simulink model "Snake_Robot_Head_Control"  (R2023a)
settings: Solver=ode23tb  StartTime=0.0  StopTime=2000  FixedStep=0.001  RelTol=1e-3
values from neighbouring files (symbols this model uses):
  cn = 5    [parameters_Robot_control.m]
  ct = 1    [parameters_Robot_control.m]
undefined symbols (not defined in the file or in its folder): X, Y, Z
libraries: nesl_utility x85, sm_lib x49
(part 3 of 3)

== system Snake_Robot_Head_Control/SnakeRobot/Link8 ==
  Brick Solid : sm_lib/Body Elements/Brick Solid  GraphicAmbientColor=[0.15 0.15 0.15 1.0]  BasedOnType=Mass  BrickDimensions=[180 80 80]  BrickDimensionsUnits=mm  CenterOfMass=[0 0 0]  CenterOfMassUnits=m  GraphicDiffuseColor=[0.5 0.5 0.5]  Density=1000  DensityUnits=kg/m^3  DoExposeReferenceFrame=on  GraphicEmissiveColor=[0.0 0.0 0.0 1.0]  ExportEntireGeometry=off  SerializedFrames=<Frames><Frame><Id>Frame1</Id><Value><Name>nextlink</Name><Origin><Source>GeometricFeature</Source><FeatureName>+x surface</FeatureName></Origin><PrimaryAxis><DefinedDirection>+Z</DefinedDirection><Source>ReferenceFrame</Source><SourceDirection>+Z</SourceDirection><FeatureName></FeatureName></PrimaryAxis><SecondaryAxis><DefinedDirection>+X</DefinedDirection><Source>ReferenceFrame</Source><SourceDirection>+X</SourceDirection><FeatureName></FeatureName></SecondaryAxis></Value></Frame><Frame><Id>Frame2</Id><Value><Name>P_link</Name><Origin><Source>GeometricFeature</Source><FeatureName>-x surface</FeatureName></Origin><PrimaryAxis><DefinedDirection>+Z</DefinedDirection><Source>ReferenceFrame</Source><SourceDirection>+Z</SourceDirection><FeatureName></FeatureName></PrimaryAxis><SecondaryAxis><DefinedDirection>+X</DefinedDirection><Source>ReferenceFrame</Source><SourceDirection>+X</SourceDirection><FeatureName></FeatureName></SecondaryAxis></Value></Frame><Frame><Id>Frame3</Id><Value><Name>F3</Name><Origin><Source>CenterOfMassFrame</Source><FeatureName></FeatureName></Origin><PrimaryAxis><DefinedDirection>+Z</DefinedDirection><Source>ReferenceFrame</Source><SourceDirection>+Z</SourceDirection><FeatureName></FeatureName></PrimaryAxis><SecondaryAxis><DefinedDirection>+X</DefinedDirection><Source>ReferenceFrame</Source><SourceDirection>+X</SourceDirection><FeatureName></FeatureName></SecondaryAxis></Value></Frame></Frames>  MarkerShape=Sphere  MarkerSize=10  GraphicType=FromGeometry  InertiaType=CalculateFromGeometry  Mass=0.9047  MassUnits=kg  MomentsOfInertia=[1 1 1]  MomentsOfInertiaUnits=kg*m^2  GraphicOpacity=1.0  ProductsOfInertia=[0 0 0]  ProductsOfInertiaUnits=kg*m^2  GraphicShininess=75  GraphicSpecularColor=[0.5 0.5 0.5 1.0]  GraphicVisPropType=SimpleVisualProperties
  Constant : Constant  Value=ct
  Constant1 : Constant  Value=cn
  Integrator : Integrator
  MATLAB Function : MATLAB Function  TreatAsAtomicUnit=on
  PS-Simulink Converter : nesl_utility/PS-Simulink Converter  PhysicalDomain=network_engine_domain  SubClassName=ps_output  LeftPortType=input  RightPortType=output  PseudoPeriodic=off  Frequencies=[]  VectorFormat=inherit  Unit=inherit  AffineConversion=off
  PS-Simulink Converter1 : nesl_utility/PS-Simulink Converter  PhysicalDomain=network_engine_domain  SubClassName=ps_output  LeftPortType=input  RightPortType=output  PseudoPeriodic=off  Frequencies=[]  VectorFormat=inherit  Unit=inherit  AffineConversion=off
  PS-Simulink Converter2 : nesl_utility/PS-Simulink Converter  PhysicalDomain=network_engine_domain  SubClassName=ps_output  LeftPortType=input  RightPortType=output  PseudoPeriodic=off  Frequencies=[]  VectorFormat=inherit  Unit=inherit  AffineConversion=off
  Planar Joint : sm_lib/Joints/Planar Joint  JointMode=Normal  SenseConstraintForce=off  SenseConstraintForceX=off  SenseConstraintForceY=off  SenseConstraintForceZ=off  SenseConstraintTorque=off  SenseConstraintTorqueX=off  SenseConstraintTorqueY=off  SenseConstraintTorqueZ=off  SenseTotalForce=off  SenseTotalForceX=off  SenseTotalForceY=off  SenseTotalForceZ=off  SenseTotalTorque=off  SenseTotalTorqueX=off  SenseTotalTorqueY=off  SenseTotalTorqueZ=off  CompositeWrenchDir=FollowerOnBase  CompositeWrenchFrame=BaseFrame  PxEquilibriumPosition=0  PxEquilibriumPositionUnits=m  PxSpringStiffness=0  PxSpringStiffnessUnits=N/m  PxDampingCoefficient=0  PxDampingCoefficientUnits=N/(m/s)  PxTorqueActuationMode=InputTorque  PxMotionActuationMode=ComputedMotion  PxSensePosition=off  PxSenseVelocity=off  PxSenseAcceleration=off  PxSenseTorqueForce=off  PxSenseLowerLimitTorqueForce=off  PxSenseUpperLimitTorqueForce=off  PxLowerLimitSpecify=off  PxLowerLimitBound=-1  PxLowerLimitBoundUnits=m  PxLowerLimitStiffness=1e6  PxLowerLimitStiffnessUnits=N/m  PxLowerLimitDamping=1e3  PxLowerLimitDampingUnits=N/(m/s)  PxLowerLimitTransitionRegionWidth=1e-4  PxLowerLimitTransitionRegionWidthUnits=m  PxUpperLimitSpecify=off  PxUpperLimitBound=1  PxUpperLimitBoundUnits=m  PxUpperLimitStiffness=1e6  PxUpperLimitStiffnessUnits=N/m  PxUpperLimitDamping=1e3  PxUpperLimitDampingUnits=N/(m/s)  PxUpperLimitTransitionRegionWidth=1e-4  PxUpperLimitTransitionRegionWidthUnits=m  PxPositionTargetSpecify=off  PxPositionTargetPriority=High  PxPositionTargetValue=0  PxPositionTargetValueUnits=m  PxVelocityTargetSpecify=off  PxVelocityTargetPriority=High  PxVelocityTargetValue=0  PxVelocityTargetValueUnits=m/s  PyEquilibriumPosition=0  PyEquilibriumPositionUnits=m  PySpringStiffness=0  PySpringStiffnessUnits=N/m  PyDampingCoefficient=0  PyDampingCoefficientUnits=N/(m/s)  PyTorqueActuationMode=InputTorque  PyMotionActuationMode=ComputedMotion  PySensePosition=off  PySenseVelocity=off  PySenseAcceleration=off  PySenseTorqueForce=off  PySenseLowerLimitTorqueForce=off  PySenseUpperLimitTorqueForce=off  PyLowerLimitSpecify=off  PyLowerLimitBound=-1  PyLowerLimitBoundUnits=m  PyLowerLimitStiffness=1e6  PyLowerLimitStiffnessUnits=N/m  PyLowerLimitDamping=1e3  PyLowerLimitDampingUnits=N/(m/s)  PyLowerLimitTransitionRegionWidth=1e-4  PyLowerLimitTransitionRegionWidthUnits=m  PyUpperLimitSpecify=off  PyUpperLimitBound=1  PyUpperLimitBoundUnits=m  PyUpperLimitStiffness=1e6  PyUpperLimitStiffnessUnits=N/m  PyUpperLimitDamping=1e3  PyUpperLimitDampingUnits=N/(m/s)  PyUpperLimitTransitionRegionWidth=1e-4  PyUpperLimitTransitionRegionWidthUnits=m  PyPositionTargetSpecify=off  PyPositionTargetPriority=High  PyPositionTargetValue=0  PyPositionTargetValueUnits=m  PyVelocityTargetSpecify=off  PyVelocityTargetPriority=High  PyVelocityTargetValue=0  PyVelocityTargetValueUnits=m/s  RzEquilibriumPosition=0  RzEquilibriumPositionUnits=deg  RzSpringStiffness=0  RzSpringStiffnessUnits=N*m/deg  RzDampingCoefficient=0  RzDampingCoefficientUnits=N*m/(deg/s)  RzTorqueActuationMode=NoTorque  RzMotionActuationMode=ComputedMotion  RzSensePosition=off  RzSenseVelocity=off  RzSenseAcceleration=off  RzSenseTorqueForce=off  RzSenseLowerLimitTorqueForce=off  RzSenseUpperLimitTorqueForce=off  RzLowerLimitSpecify=off  RzLowerLimitBound=-90  RzLowerLimitBoundUnits=deg  RzLowerLimitStiffness=1e4  RzLowerLimitStiffnessUnits=N*m/deg  RzLowerLimitDamping=10  RzLowerLimitDampingUnits=N*m/(deg/s)  RzLowerLimitTransitionRegionWidth=0.1  RzLowerLimitTransitionRegionWidthUnits=deg  RzUpperLimitSpecify=off  RzUpperLimitBound=90  RzUpperLimitBoundUnits=deg  RzUpperLimitStiffness=1e4  RzUpperLimitStiffnessUnits=N*m/deg  RzUpperLimitDamping=10  RzUpperLimitDampingUnits=N*m/(deg/s)  RzUpperLimitTransitionRegionWidth=0.1  RzUpperLimitTransitionRegionWidthUnits=deg  RzPositionTargetSpecify=off  RzPositionTargetPriority=High  RzPositionTargetValue=0  RzPositionTargetValueUnits=deg  RzVelocityTargetSpecify=off  RzVelocityTargetPriority=High  RzVelocityTargetValue=0  RzVelocityTargetValueUnits=deg/s
  Simulink-PS Converter : nesl_utility/Simulink-PS Converter  PhysicalDomain=network_engine_domain  SubClassName=ps_input  LeftPortType=input  RightPortType=output  PseudoPeriodic=off  Frequencies=[]  NoiseDistribution=none  NoiseParameters=[]  Unit=1  AffineConversion=off  FilteringAndDerivatives=provide  SimscapeFilterOrder=1  InputFilterTimeConstant=0.001  UdotUserProvided=0
  Simulink-PS Converter1 : nesl_utility/Simulink-PS Converter  PhysicalDomain=network_engine_domain  SubClassName=ps_input  LeftPortType=input  RightPortType=output  PseudoPeriodic=off  Frequencies=[]  NoiseDistribution=none  NoiseParameters=[]  Unit=1  AffineConversion=off  FilteringAndDerivatives=provide  SimscapeFilterOrder=1  InputFilterTimeConstant=0.001  UdotUserProvided=0
  Transform Sensor : sm_lib/Frames and Transforms/Transform Sensor  MeasurementFrame=World  RotationSequence=XYX  SenseAngle=on  SenseAxis=off  SenseQ=off  SenseR=off  SenseRotationSequence=off  SenseOmegaX=off  SenseOmegaY=off  SenseOmegaZ=on  SenseQDot=off  SenseRDot=off  SenseRotationSequenceDot=off  SenseAlphaX=off  SenseAlphaY=off  SenseAlphaZ=off  SenseQDDot=off  SenseRDDot=off  SenseX=on  SenseY=on  SenseZ=off  SenseRad=off  SenseAzim=off  SenseDist=off  SenseInc=off  SenseXDot=on  SenseYDot=on  SenseZDot=off  SenseRadDot=off  SenseAzimDot=off  SenseDistDot=off  SenseIncDot=off  SenseXDDot=off  SenseYDDot=off  SenseZDDot=off  SenseRadDDot=off  SenseAzimDDot=off  SenseDistDDot=off  SenseIncDDot=off
  World Frame : sm_lib/Frames and Transforms/World Frame
  N_Link : PMIOPort  Side=Left
  G : PMIOPort  Port=2  Side=Left
  P_Link : PMIOPort  Port=3  Side=Right
  q1 : PMIOPort  Port=4  Side=Right
  dot q1 : PMIOPort  Port=5  Side=Right
  x1 : PMIOPort  Port=6  Side=Right
  y1 : PMIOPort  Port=7  Side=Right
  vx1 : PMIOPort  Port=8  Side=Right
  vy1 : PMIOPort  Port=9  Side=Right
  wires:
  MATLAB Function/1(fx) -> Simulink-PS Converter/1
  MATLAB Function/2(fy) -> Simulink-PS Converter1/1
  Constant1/1 -> MATLAB Function/4(cn)
  Constant/1 -> MATLAB Function/3(ct)
  Integrator/1 -> MATLAB Function/5(th)
  PS-Simulink Converter1/1 -> MATLAB Function/2(vy)
  PS-Simulink Converter/1 -> MATLAB Function/1(vx)
  PS-Simulink Converter2/1 -> Integrator/1
  connections:
  q1/RConn1 -- Transform Sensor/RConn2
  Simulink-PS Converter1/RConn1 -- Planar Joint/LConn3
  Brick Solid/RConn2 -- Planar Joint/RConn1
  Simulink-PS Converter/RConn1 -- Planar Joint/LConn2
  Transform Sensor/RConn6 -- PS-Simulink Converter/LConn1 -- vx1/RConn1
  Transform Sensor/RConn7 -- vy1/RConn1 -- PS-Simulink Converter1/LConn1
  Transform Sensor/RConn1 -- Brick Solid/RConn1
  World Frame/RConn1 -- Transform Sensor/LConn1
  G/RConn1 -- Planar Joint/LConn1
  N_Link/RConn1 -- Brick Solid/LConn1
  P_Link/RConn1 -- Brick Solid/LConn2
  dot q1/RConn1 -- Transform Sensor/RConn3 -- PS-Simulink Converter2/LConn1
  x1/RConn1 -- Transform Sensor/RConn4
  Transform Sensor/RConn5 -- y1/RConn1

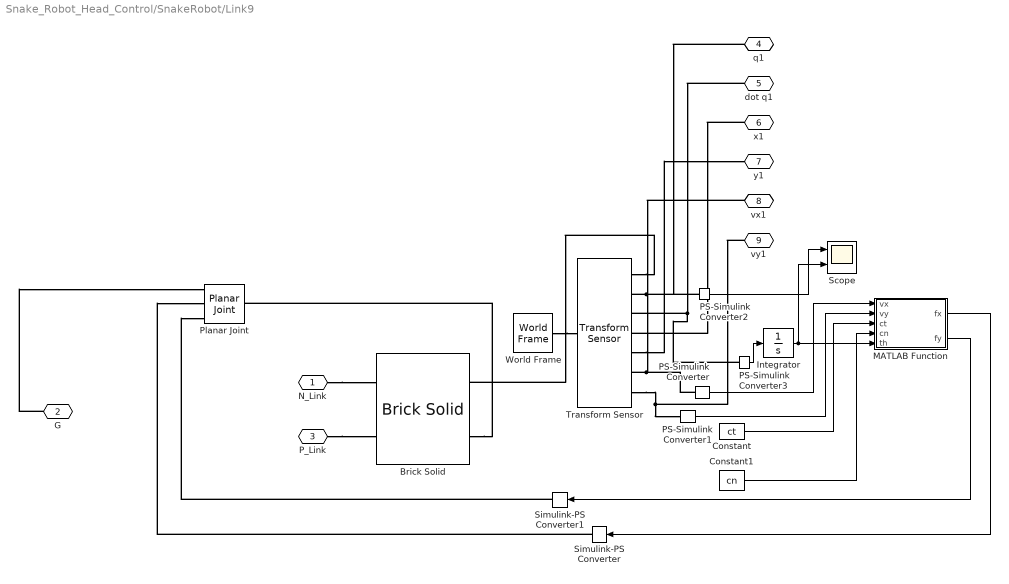
== system Snake_Robot_Head_Control/SnakeRobot/Link9 ==
  Brick Solid : sm_lib/Body Elements/Brick Solid  GraphicAmbientColor=[0.15 0.15 0.15 1.0]  BasedOnType=Mass  BrickDimensions=[180 80 80]  BrickDimensionsUnits=mm  CenterOfMass=[0 0 0]  CenterOfMassUnits=m  GraphicDiffuseColor=[0.5 0.5 0.5]  Density=1000  DensityUnits=kg/m^3  DoExposeReferenceFrame=on  GraphicEmissiveColor=[0.0 0.0 0.0 1.0]  ExportEntireGeometry=off  SerializedFrames=<Frames><Frame><Id>Frame1</Id><Value><Name>nextlink</Name><Origin><Source>GeometricFeature</Source><FeatureName>+x surface</FeatureName></Origin><PrimaryAxis><DefinedDirection>+Z</DefinedDirection><Source>ReferenceFrame</Source><SourceDirection>+Z</SourceDirection><FeatureName></FeatureName></PrimaryAxis><SecondaryAxis><DefinedDirection>+X</DefinedDirection><Source>ReferenceFrame</Source><SourceDirection>+X</SourceDirection><FeatureName></FeatureName></SecondaryAxis></Value></Frame><Frame><Id>Frame2</Id><Value><Name>P_link</Name><Origin><Source>GeometricFeature</Source><FeatureName>-x surface</FeatureName></Origin><PrimaryAxis><DefinedDirection>+Z</DefinedDirection><Source>ReferenceFrame</Source><SourceDirection>+Z</SourceDirection><FeatureName></FeatureName></PrimaryAxis><SecondaryAxis><DefinedDirection>+X</DefinedDirection><Source>ReferenceFrame</Source><SourceDirection>+X</SourceDirection><FeatureName></FeatureName></SecondaryAxis></Value></Frame><Frame><Id>Frame3</Id><Value><Name>F3</Name><Origin><Source>CenterOfMassFrame</Source><FeatureName></FeatureName></Origin><PrimaryAxis><DefinedDirection>+Z</DefinedDirection><Source>ReferenceFrame</Source><SourceDirection>+Z</SourceDirection><FeatureName></FeatureName></PrimaryAxis><SecondaryAxis><DefinedDirection>+X</DefinedDirection><Source>ReferenceFrame</Source><SourceDirection>+X</SourceDirection><FeatureName></FeatureName></SecondaryAxis></Value></Frame></Frames>  MarkerShape=Sphere  MarkerSize=10  GraphicType=FromGeometry  InertiaType=CalculateFromGeometry  Mass=0.9047  MassUnits=kg  MomentsOfInertia=[1 1 1]  MomentsOfInertiaUnits=kg*m^2  GraphicOpacity=1.0  ProductsOfInertia=[0 0 0]  ProductsOfInertiaUnits=kg*m^2  GraphicShininess=75  GraphicSpecularColor=[0.5 0.5 0.5 1.0]  GraphicVisPropType=SimpleVisualProperties
  Constant : Constant  Value=ct
  Constant1 : Constant  Value=cn
  Integrator : Integrator
  MATLAB Function : MATLAB Function  TreatAsAtomicUnit=on
  PS-Simulink Converter{,1..3} (4 alike) : nesl_utility/PS-Simulink Converter  PhysicalDomain=network_engine_domain  SubClassName=ps_output  LeftPortType=input  RightPortType=output  PseudoPeriodic=off  Frequencies=[]  VectorFormat=inherit  Unit=inherit  AffineConversion=off
  Planar Joint : sm_lib/Joints/Planar Joint  JointMode=Normal  SenseConstraintForce=off  SenseConstraintForceX=off  SenseConstraintForceY=off  SenseConstraintForceZ=off  SenseConstraintTorque=off  SenseConstraintTorqueX=off  SenseConstraintTorqueY=off  SenseConstraintTorqueZ=off  SenseTotalForce=off  SenseTotalForceX=off  SenseTotalForceY=off  SenseTotalForceZ=off  SenseTotalTorque=off  SenseTotalTorqueX=off  SenseTotalTorqueY=off  SenseTotalTorqueZ=off  CompositeWrenchDir=FollowerOnBase  CompositeWrenchFrame=BaseFrame  PxEquilibriumPosition=0  PxEquilibriumPositionUnits=m  PxSpringStiffness=0  PxSpringStiffnessUnits=N/m  PxDampingCoefficient=0  PxDampingCoefficientUnits=N/(m/s)  PxTorqueActuationMode=InputTorque  PxMotionActuationMode=ComputedMotion  PxSensePosition=off  PxSenseVelocity=off  PxSenseAcceleration=off  PxSenseTorqueForce=off  PxSenseLowerLimitTorqueForce=off  PxSenseUpperLimitTorqueForce=off  PxLowerLimitSpecify=off  PxLowerLimitBound=-1  PxLowerLimitBoundUnits=m  PxLowerLimitStiffness=1e6  PxLowerLimitStiffnessUnits=N/m  PxLowerLimitDamping=1e3  PxLowerLimitDampingUnits=N/(m/s)  PxLowerLimitTransitionRegionWidth=1e-4  PxLowerLimitTransitionRegionWidthUnits=m  PxUpperLimitSpecify=off  PxUpperLimitBound=1  PxUpperLimitBoundUnits=m  PxUpperLimitStiffness=1e6  PxUpperLimitStiffnessUnits=N/m  PxUpperLimitDamping=1e3  PxUpperLimitDampingUnits=N/(m/s)  PxUpperLimitTransitionRegionWidth=1e-4  PxUpperLimitTransitionRegionWidthUnits=m  PxPositionTargetSpecify=off  PxPositionTargetPriority=High  PxPositionTargetValue=0  PxPositionTargetValueUnits=m  PxVelocityTargetSpecify=off  PxVelocityTargetPriority=High  PxVelocityTargetValue=0  PxVelocityTargetValueUnits=m/s  PyEquilibriumPosition=0  PyEquilibriumPositionUnits=m  PySpringStiffness=0  PySpringStiffnessUnits=N/m  PyDampingCoefficient=0  PyDampingCoefficientUnits=N/(m/s)  PyTorqueActuationMode=InputTorque  PyMotionActuationMode=ComputedMotion  PySensePosition=off  PySenseVelocity=off  PySenseAcceleration=off  PySenseTorqueForce=off  PySenseLowerLimitTorqueForce=off  PySenseUpperLimitTorqueForce=off  PyLowerLimitSpecify=off  PyLowerLimitBound=-1  PyLowerLimitBoundUnits=m  PyLowerLimitStiffness=1e6  PyLowerLimitStiffnessUnits=N/m  PyLowerLimitDamping=1e3  PyLowerLimitDampingUnits=N/(m/s)  PyLowerLimitTransitionRegionWidth=1e-4  PyLowerLimitTransitionRegionWidthUnits=m  PyUpperLimitSpecify=off  PyUpperLimitBound=1  PyUpperLimitBoundUnits=m  PyUpperLimitStiffness=1e6  PyUpperLimitStiffnessUnits=N/m  PyUpperLimitDamping=1e3  PyUpperLimitDampingUnits=N/(m/s)  PyUpperLimitTransitionRegionWidth=1e-4  PyUpperLimitTransitionRegionWidthUnits=m  PyPositionTargetSpecify=off  PyPositionTargetPriority=High  PyPositionTargetValue=0  PyPositionTargetValueUnits=m  PyVelocityTargetSpecify=off  PyVelocityTargetPriority=High  PyVelocityTargetValue=0  PyVelocityTargetValueUnits=m/s  RzEquilibriumPosition=0  RzEquilibriumPositionUnits=deg  RzSpringStiffness=0  RzSpringStiffnessUnits=N*m/deg  RzDampingCoefficient=0  RzDampingCoefficientUnits=N*m/(deg/s)  RzTorqueActuationMode=NoTorque  RzMotionActuationMode=ComputedMotion  RzSensePosition=off  RzSenseVelocity=off  RzSenseAcceleration=off  RzSenseTorqueForce=off  RzSenseLowerLimitTorqueForce=off  RzSenseUpperLimitTorqueForce=off  RzLowerLimitSpecify=off  RzLowerLimitBound=-90  RzLowerLimitBoundUnits=deg  RzLowerLimitStiffness=1e4  RzLowerLimitStiffnessUnits=N*m/deg  RzLowerLimitDamping=10  RzLowerLimitDampingUnits=N*m/(deg/s)  RzLowerLimitTransitionRegionWidth=0.1  RzLowerLimitTransitionRegionWidthUnits=deg  RzUpperLimitSpecify=off  RzUpperLimitBound=90  RzUpperLimitBoundUnits=deg  RzUpperLimitStiffness=1e4  RzUpperLimitStiffnessUnits=N*m/deg  RzUpperLimitDamping=10  RzUpperLimitDampingUnits=N*m/(deg/s)  RzUpperLimitTransitionRegionWidth=0.1  RzUpperLimitTransitionRegionWidthUnits=deg  RzPositionTargetSpecify=off  RzPositionTargetPriority=High  RzPositionTargetValue=0  RzPositionTargetValueUnits=deg  RzVelocityTargetSpecify=off  RzVelocityTargetPriority=High  RzVelocityTargetValue=0  RzVelocityTargetValueUnits=deg/s
  Scope : Scope  NumInputPorts=2
  Simulink-PS Converter : nesl_utility/Simulink-PS Converter  PhysicalDomain=network_engine_domain  SubClassName=ps_input  LeftPortType=input  RightPortType=output  PseudoPeriodic=off  Frequencies=[]  NoiseDistribution=none  NoiseParameters=[]  Unit=1  AffineConversion=off  FilteringAndDerivatives=provide  SimscapeFilterOrder=1  InputFilterTimeConstant=0.001  UdotUserProvided=0
  Simulink-PS Converter1 : nesl_utility/Simulink-PS Converter  PhysicalDomain=network_engine_domain  SubClassName=ps_input  LeftPortType=input  RightPortType=output  PseudoPeriodic=off  Frequencies=[]  NoiseDistribution=none  NoiseParameters=[]  Unit=1  AffineConversion=off  FilteringAndDerivatives=provide  SimscapeFilterOrder=1  InputFilterTimeConstant=0.001  UdotUserProvided=0
  Transform Sensor : sm_lib/Frames and Transforms/Transform Sensor  MeasurementFrame=World  RotationSequence=ZYX  SenseAngle=on  SenseAxis=off  SenseQ=off  SenseR=off  SenseRotationSequence=off  SenseOmegaX=off  SenseOmegaY=off  SenseOmegaZ=on  SenseQDot=off  SenseRDot=off  SenseRotationSequenceDot=off  SenseAlphaX=off  SenseAlphaY=off  SenseAlphaZ=off  SenseQDDot=off  SenseRDDot=off  SenseX=on  SenseY=on  SenseZ=off  SenseRad=off  SenseAzim=off  SenseDist=off  SenseInc=off  SenseXDot=on  SenseYDot=on  SenseZDot=off  SenseRadDot=off  SenseAzimDot=off  SenseDistDot=off  SenseIncDot=off  SenseXDDot=off  SenseYDDot=off  SenseZDDot=off  SenseRadDDot=off  SenseAzimDDot=off  SenseDistDDot=off  SenseIncDDot=off
  World Frame : sm_lib/Frames and Transforms/World Frame
  N_Link : PMIOPort  Side=Left
  G : PMIOPort  Port=2  Side=Left
  P_Link : PMIOPort  Port=3  Side=Right
  q1 : PMIOPort  Port=4  Side=Right
  dot q1 : PMIOPort  Port=5  Side=Right
  x1 : PMIOPort  Port=6  Side=Right
  y1 : PMIOPort  Port=7  Side=Right
  vx1 : PMIOPort  Port=8  Side=Right
  vy1 : PMIOPort  Port=9  Side=Right
  wires:
  MATLAB Function/1(fx) -> Simulink-PS Converter/1
  MATLAB Function/2(fy) -> Simulink-PS Converter1/1
  Constant1/1 -> MATLAB Function/4(cn)
  Constant/1 -> MATLAB Function/3(ct)
  PS-Simulink Converter2/1 -> Scope/1
  PS-Simulink Converter1/1 -> MATLAB Function/2(vy)
  PS-Simulink Converter/1 -> MATLAB Function/1(vx)
  PS-Simulink Converter3/1 -> Integrator/1
  Integrator/1 -> Scope/2, MATLAB Function/5(th)
  connections:
  Transform Sensor/RConn2 -- PS-Simulink Converter2/LConn1 -- q1/RConn1
  Simulink-PS Converter1/RConn1 -- Planar Joint/LConn3
  Brick Solid/RConn2 -- Planar Joint/RConn1
  Simulink-PS Converter/RConn1 -- Planar Joint/LConn2
  Transform Sensor/RConn6 -- PS-Simulink Converter/LConn1 -- vx1/RConn1
  Transform Sensor/RConn7 -- vy1/RConn1 -- PS-Simulink Converter1/LConn1
  Transform Sensor/RConn1 -- Brick Solid/RConn1
  World Frame/RConn1 -- Transform Sensor/LConn1
  G/RConn1 -- Planar Joint/LConn1
  N_Link/RConn1 -- Brick Solid/LConn1
  P_Link/RConn1 -- Brick Solid/LConn2
  dot q1/RConn1 -- PS-Simulink Converter3/LConn1 -- Transform Sensor/RConn3
  x1/RConn1 -- Transform Sensor/RConn4
  Transform Sensor/RConn5 -- y1/RConn1

== matlab function Snake_Robot_Head_Control/SnakeRobot/Link7/MATLAB Function ==
  data: vx input; fx output; vy input; ct input; cn input; th input; fy output
function [fx,fy] = fcn(vx,vy,ct,cn,th)
fx = -(ct*(cos(th))^2+cn*(sin(th))^2)*vx-((ct-cn)*sin(th)*cos(th))*vy;
fy = -((ct-cn)*sin(th)*cos(th))*vx-(ct*(sin(th))^2+cn*(cos(th))^2)*vy;
% fx = -ct*vx;
% fy = -cn*vy;
end

== matlab function Snake_Robot_Head_Control/SnakeRobot/Link8/MATLAB Function ==
  data: vx input; fx output; vy input; ct input; cn input; th input; fy output
function [fx,fy] = fcn(vx,vy,ct,cn,th)
fx = -(ct*(cos(th))^2+cn*(sin(th))^2)*vx-((ct-cn)*sin(th)*cos(th))*vy;
fy = -((ct-cn)*sin(th)*cos(th))*vx-(ct*(sin(th))^2+cn*(cos(th))^2)*vy;
% fx = -ct*vx;
% fy = -cn*vy;
end

== matlab function Snake_Robot_Head_Control/SnakeRobot/Link9/MATLAB Function ==
  data: vx input; fx output; vy input; ct input; cn input; th input; fy output
function [fx,fy] = fcn(vx,vy,ct,cn,th)
fx = -(ct*(cos(th))^2+cn*(sin(th))^2)*vx-((ct-cn)*sin(th)*cos(th))*vy+0.02;
fy = -((ct-cn)*sin(th)*cos(th))*vx-(ct*(sin(th))^2+cn*(cos(th))^2)*vy+0.002*sign(-th);
% fx = -ct*vx;
% fy = -cn*vy;
end

== matlab function Snake_Robot_Head_Control/wave generation1 ==
  data: phi input; dphi input; phir output; t input; dphir output
function [phir,dphir]   = fcn(phi,dphi,t)
n = 9;
alpha = pi/6;
delta =pi/3;
gamma = 1*t;
phi1 = alpha*sin(gamma+0*delta)+phi;
phi2 = alpha*sin(gamma+1*delta);
phi3 = alpha*sin(gamma+2*delta);
phi4 = alpha*sin(gamma+3*delta);
phi5 = alpha*sin(gamma+4*delta);
phi6 = alpha*sin(gamma+5*delta);
phi7 = alpha*sin(gamma+6*delta);
phi8 = alpha*sin(gamma+7*delta)+phi;
phir = [phi1,phi2,phi3,phi4,phi5,phi6,phi7,phi8]';

dphi1 = alpha*cos(gamma+0*delta)+dphi;
dphi2 = alpha*cos(gamma+1*delta);
dphi3 = alpha*cos(gamma+2*delta);
dphi4 = alpha*cos(gamma+3*delta);
dphi5 = alpha*cos(gamma+4*delta);
dphi6 = alpha*cos(gamma+5*delta);
dphi7 = alpha*cos(gamma+6*delta);
dphi8 = alpha*cos(gamma+7*delta)+dphi;

dphir = [dphi1,dphi2,dphi3,dphi4,dphi5,dphi6,dphi7,dphi8]';

% ddphi1 = -alpha*sin(gamma+0*delta)+d_gamma*dphi1+dd_gamma*phi1+d_gamma*alpha*cos(gamma+0*delta)+ddphi;
% ddphi2 = -alpha*sin(gamma+1*delta)+d_gamma*dphi2+dd_gamma*phi2+d_gamma*alpha*cos(gamma+1*delta)+ddphi;
% ddphi3 = -alpha*sin(gamma+2*delta)+d_gamma*dphi3+dd_gamma*phi3+d_gamma*alpha*cos(gamma+2*delta)+ddphi;
% ddphi4 = -alpha*sin(gamma+3*delta)+d_gamma*dphi4+dd_gamma*phi4+d_gamma*alpha*cos(gamma+3*delta)+ddphi;
% ddphi5 = -alpha*sin(gamma+4*delta)+d_gamma*dphi5+dd_gamma*phi5+d_gamma*alpha*cos(gamma+4*delta)+ddphi;
% ddphi6 = -alpha*sin(gamma+5*delta)+d_gamma*dphi6+dd_gamma*phi6+d_gamma*alpha*cos(gamma+5*delta)+ddphi;
% ddphi7 = -alpha*sin(gamma+6*delta)+d_gamma*dphi7+dd_gamma*phi7+d_gamma*alpha*cos(gamma+6*delta)+ddphi;
% ddphi8 = -alpha*sin(gamma+7*delta)+d_gamma*dphi8+dd_gamma*phi8+d_gamma*alpha*cos(gamma+7*delta)+ddphi;
% 
% ddphir = [ddphi1,ddphi2,ddphi3,ddphi4,ddphi5,ddphi6,ddphi7,ddphi8]';

== matlab function Snake_Robot_Head_Control/Reference Signal/control input ==
  data: th input; u output; ph_G input; ph_0 input; dph_G input; d_gamma input; dph_0 input; dth input; ie input; phi output; g output; Er output
function [u,phi,g,Er] = fcn(th,ph_G,ph_0,dph_G,d_gamma,dph_0,dth,ie)
n = 9;
% m = 0.9047;
% l = 0.09;
% J = 1/3*m*l^2;
% % ct = 4.45;
% % cn = 17.3;
% % lambda2 = 0.015;
% % lambda3 = 1.2*10^-3;
% % ct = 6.5;
% % cn = 16.50;
% lambda2 = 0.016;
% lambda3 = 7*10^-4;
% ct = 6.5;
% cn = 17.50;
% L2 = lambda2*eye(n);
% L3 = lambda3*eye(n);
% % vcx = -0.01;
% % vcy = 0.01;
% vc =[0,0]';
% vcx = vc(1);
% vcy = vc(2);
% 
A = [1 1 0 0 0 0 0 0 0;
    0 1 1 0 0 0 0 0 0;
    0 0 1 1 0 0 0 0 0;
    0 0 0 1 1 0 0 0 0;
    0 0 0 0 1 1 0 0 0;
    0 0 0 0 0 1 1 0 0;
    0 0 0 0 0 0 1 1 0;
    0 0 0 0 0 0 0 1 1];
D = [1 -1 0 0 0 0 0 0 0;
    0 1 -1 0 0 0 0 0 0;
    0 0 1 -1 0 0 0 0 0;
    0 0 0 1 -1 0 0 0 0;
    0 0 0 0 1 -1 0 0 0;
    0 0 0 0 0 1 -1 0 0;
    0 0 0 0 0 0 1 -1 0;
    0 0 0 0 0 0 0 1 -1];
e = ones(n,1);
E = [e zeros(n,1);zeros(n,1) e];
H = ones(n-1);
H = triu(H);
H = [H;zeros(1,n-1)];
% 
% sinth = [sin(th(1)),sin(th(2)),sin(th(3)),sin(th(4)),sin(th(5)),sin(th(6)),sin(th(7)),sin(th(8)),sin(th(9))]';
% costh = [cos(th(1)),cos(th(2)),cos(th(3)),cos(th(4)),cos(th(5)),cos(th(6)),cos(th(7)),cos(th(8)),cos(th(9))]';
% Sth = diag(sinth);
% Cth = diag(costh);
% 
% Vx = e*vcx;
% Vy = e*vcy;
% 
% V = A'*inv(D*D')*A;
% K = A'*inv(D*D')*D;
% Vr = [Cth, Sth;-Sth,Cth]*[(l*K'*Sth*dth+e*dpx-Vx);(-l*K'*Cth*dth+e*dpy-Vy)];
% 
% SCth = [K'*Sth;-K'*Cth];
% Mth = J*eye(n) + m*l^2*Sth*V*Sth + m*l^2*Cth*V*Cth;
% Wth = m*l^2*Sth*V*Cth - m*l^2*Cth*V*Sth;
% Qth = -[ct*Cth*Cth+cn*Sth*Sth, (ct-cn)*Sth*Cth;
%     (ct-cn)*Sth*Cth, ct*Sth*Sth+cn*Cth*Cth];
% vr = [dpx;dpy]-vc;
% Fdnl = -[ct*Cth, cn*Sth;
%     ct*Cth, cn*Cth]*diag(sign([Vr(1:n);Vr(n+1:2*n)]))*diag([Vr(1:n);Vr(n+1:2*n)])*[Vr(1:n);Vr(n+1:2*n)];
% 
% Fd = l*Qth*SCth*dth + Qth*E*vr + Fdnl;

Kp = 20;
Kd = 5;
ki=10;
%kuG = 0.1;
%kup = 0.1;
b = ones(n-1,1);
Er = (D*th - ph_G -b*ph_0);
%b=[zeros(7,1);ones(1,1)];
u = -Kp*Er - Kd*(D*dth - dph_G*d_gamma - b*dph_0)-ki*ie;
% Mp = inv(Mth);
% u = inv(D*Mp*D')*(D*Mp*Wth*diag(dth)*dth + D*Mp*L2*dth + D*Mp*L3*diag(abs(dth))*dth - l*D*Mp*SCth'*Fd + ddph_G*d_gamma^2 + dph_G*u_G + b*u_ph - Kp*(D*th - ph_G - b*ph_0) - Kd*(D*dth - dph_G*d_gamma - b*dph_0));
% u1 = u(1);
% u2 = u(2);
% u3 = u(3);
% u4 = u(4);
% u5 = u(5);
% u6 = u(6);
% u7 = u(7);
% u8 = u(8);
% uf = [u1,u2,u3,u4,u5,u6,u7,u8]';
phi = D*th;
g = D*th-ph_G-b*ph_0;

== matlab function Snake_Robot_Head_Control/Head Control ==
  data: dthn_e input; thn_e input; ph_0 input; dph_0 input; u_ph output
function u_ph = fcn(dthn_e,thn_e,ph_0,dph_0)

epsilon = 10;
kn = 0.01;
k1 = 0.01;
k2 = 0.01;
u_ph = -(dthn_e + kn*thn_e)/(epsilon) - k1*ph_0 - k2*dph_0;

== matlab function Snake_Robot_Head_Control/PD Control/MATLAB Function ==
  data: phir input; u output; dphir input; Q input; dQ input
function u = fcn(phir,dphir,Q,dQ)
kp = 40;
kd = 10;
u = kp*(phir-Q)+kd*(dphir-dQ);

== matlab function Snake_Robot_Head_Control/SnakeRobot/Link2/MATLAB Function ==
  data: vx input; fx output; vy input; ct input; cn input; th input; fy output
function [fx,fy] = fcn(vx,vy,ct,cn,th)
fx = -(ct*(cos(th))^2+cn*(sin(th))^2)*vx-((ct-cn)*sin(th)*cos(th))*vy;
fy = -((ct-cn)*sin(th)*cos(th))*vx-(ct*(sin(th))^2+cn*(cos(th))^2)*vy;
% fx = -ct*vx;
% fy = -cn*vy;
end

== matlab function Snake_Robot_Head_Control/SnakeRobot/Link1/MATLAB Function ==
  data: vx input; fx output; vy input; ct input; cn input; th input; fy output
function [fx,fy] = fcn(vx,vy,ct,cn,th)
fx = -(ct*(cos(th))^2+cn*(sin(th))^2)*vx-((ct-cn)*sin(th)*cos(th))*vy;
fy = -((ct-cn)*sin(th)*cos(th))*vx-(ct*(sin(th))^2+cn*(cos(th))^2)*vy;
% fx = -ct*vx;
% fy = -cn*vy;
end

== matlab function Snake_Robot_Head_Control/SnakeRobot/Link3/MATLAB Function ==
  data: vx input; fx output; vy input; ct input; cn input; th input; fy output
function [fx,fy] = fcn(vx,vy,ct,cn,th)
fx = -(ct*(cos(th))^2+cn*(sin(th))^2)*vx-((ct-cn)*sin(th)*cos(th))*vy;
fy = -((ct-cn)*sin(th)*cos(th))*vx-(ct*(sin(th))^2+cn*(cos(th))^2)*vy;
% fx = -ct*vx;
% fy = -cn*vy;
end

== matlab function Snake_Robot_Head_Control/SnakeRobot/Link4/MATLAB Function ==
  data: vx input; fx output; vy input; ct input; cn input; th input; fy output
function [fx,fy] = fcn(vx,vy,ct,cn,th)
fx = -(ct*(cos(th))^2+cn*(sin(th))^2)*vx-((ct-cn)*sin(th)*cos(th))*vy;
fy = -((ct-cn)*sin(th)*cos(th))*vx-(ct*(sin(th))^2+cn*(cos(th))^2)*vy;
% fx = -ct*vx;
% fy = -cn*vy;
end

== matlab function Snake_Robot_Head_Control/SnakeRobot/Link5/MATLAB Function ==
  data: vx input; fx output; vy input; ct input; cn input; th input; fy output
function [fx,fy] = fcn(vx,vy,ct,cn,th)
fx = -(ct*(cos(th))^2+cn*(sin(th))^2)*vx-((ct-cn)*sin(th)*cos(th))*vy;
fy = -((ct-cn)*sin(th)*cos(th))*vx-(ct*(sin(th))^2+cn*(cos(th))^2)*vy;
% fx = -ct*vx;
% fy = -cn*vy;
end

== matlab function Snake_Robot_Head_Control/SnakeRobot/Link6/MATLAB Function ==
  data: vx input; fx output; vy input; ct input; cn input; th input; fy output
function [fx,fy] = fcn(vx,vy,ct,cn,th)
fx = -(ct*(cos(th))^2+cn*(sin(th))^2)*vx-((ct-cn)*sin(th)*cos(th))*vy;
fy = -((ct-cn)*sin(th)*cos(th))*vx-(ct*(sin(th))^2+cn*(cos(th))^2)*vy;
% fx = -ct*vx;
% fy = -cn*vy;
end
